simulink model "double_mass_spring_damper"  (R2019b)
settings: Solver=FixedStepAuto  StartTime=0.0  StopTime=50  FixedStep=0.01  RelTol=1e-3
values from neighbouring files (symbols this model uses):
  A = [0.969169519504925  -0.246386829627017;  0.049277365925403  0.993808202467626]    [DMDc_MW.m]    (also in DMDc_param_sweep.m = real(A); EKF_msd_estimator.m = [0, 1; -k/m, -b/m]; HAVOK.m = AB(:,1:q*m); HAVOK_param_sweep.m = real(A))
  B = [0.049277365925403; 0.001238359506475]    [DMDc_MW.m]    (also in DMDc_param_sweep.m = AB(:,(q*m+1):end); EKF_estimator.m = zeros(nx,1); EKF_msd_estimator.m = [0; 1/m]; HAVOK.m = AB(:,(q*m+1):end))
  C = [0 1]    [DMDc_MW.m]    (also in EKF_estimator.m = eye(6); EKF_msd_estimator.m = [1, 0]; KF_estimator.m = [1, 0]; LS.m)
  nu = size_B(2)    [DMDc_MW.m]    (also in EKF_msd_estimator.m = 1; LS.m; Linear_regression_state_estimator.m = 2; cart_pend_DMD_script.m)
  nx = size_B(1)    [DMDc_MW.m]    (also in EKF_msd_estimator.m = 2; LS.m; Linear_regression_state_estimator.m = 4; cart_pend_DMD_script.m)
  x0 = [0; 0; 0; 0; 0; 1]    [EKF_estimator.m]    (also in EKF_msd_estimator.m = [0; 0]; HAVOK.m = [0.5; 0]; KF_estimator.m = [0; 0]; Linear_regression_state_estimator.m = [0;0;0;0])
settings Model: Creator=Murray  LastModifiedBy=Murray

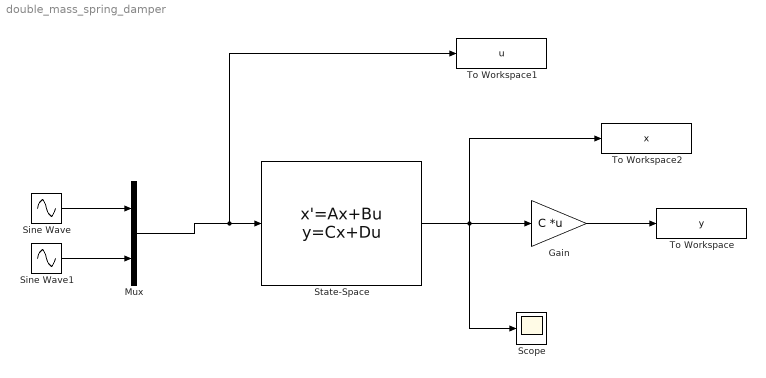
== system double_mass_spring_damper ==
  Gain : Gain  Gain=C  Multiplication=Matrix(K*u)
  Mux : Mux  Inputs=2
  Scope : Scope
  Sine Wave : Sin  SampleTime=0
  Sine Wave1 : Sin  Amplitude=2  Frequency=0.8  SampleTime=0
  State-Space : StateSpace  A=A  B=B  C=eye(nx)  D=zeros(nx,nu)  InitialCondition=x0
  To Workspace : ToWorkspace  VariableName=y  SaveFormat=Timeseries  SampleTime=-1
  To Workspace1 : ToWorkspace  VariableName=u  SaveFormat=Timeseries  SampleTime=-1
  To Workspace2 : ToWorkspace  VariableName=x  SaveFormat=Timeseries  SampleTime=-1
  wires:
  Sine Wave1/1 -> Mux/2
  Sine Wave/1 -> Mux/1
  Mux/1 -> To Workspace1/1, State-Space/1
  State-Space/1 -> To Workspace2/1, Scope/1, Gain/1
  Gain/1 -> To Workspace/1
